simulink subsystem "Vehicle_Forces_Moments"  (R2025b)
settings: Solver=VariableStepAuto  StartTime=0.0  StopTime=10.0  RelTol=1e-3
undefined symbols (not defined in the file): ActTC
libraries: aerolibactuator x2
settings Model: Creator=cdriggs  LastModifiedBy=Ky Bui

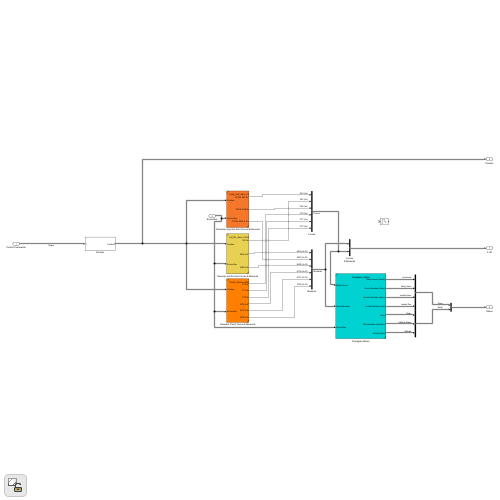
[thumbnail: Simulink's stored preview of the top-level diagram]
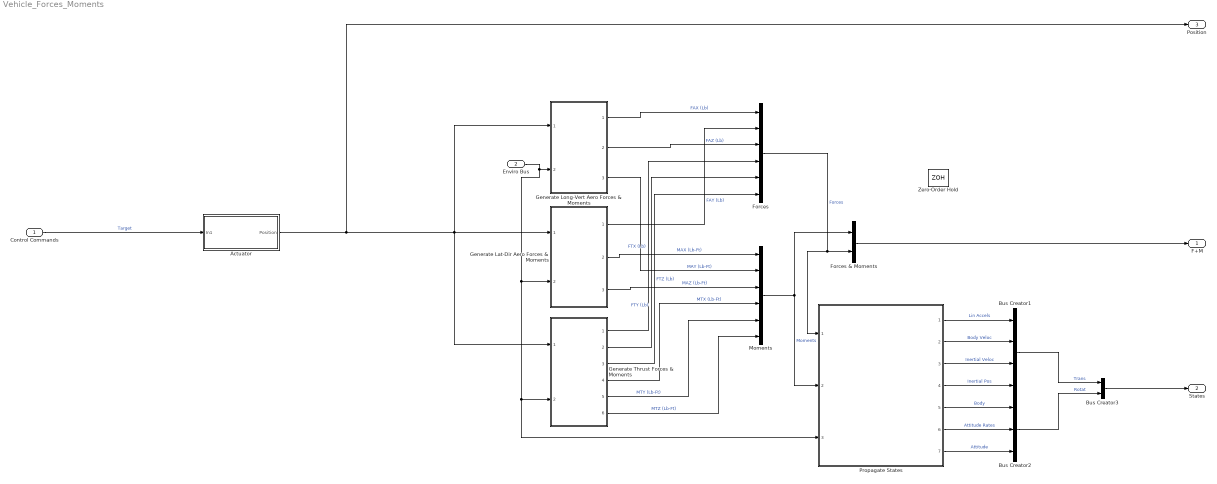
== system Vehicle_Forces_Moments ==
  Control Commands : Inport
  Enviro Bus : Inport  Port=2
  Actuator : Subsystem
  Bus Creator1 : BusCreator  Inputs=4
  Bus Creator2 : BusCreator  Inputs=3
  Bus Creator3 : BusCreator  Inputs=2
  Forces : BusCreator  Inputs=6
  Forces & Moments : BusCreator  Inputs=2
  Generate Lat-Dir Aero Forces & Moments : Subsystem  ReferencedSubsystem=Lat_Dir_Aero_Forces_Moments
  Generate Long-Vert Aero Forces & Moments : Subsystem  ReferencedSubsystem=Long_Vert_Aero_Forces_Moments
  Generate Thrust Forces & Moments : Subsystem  ReferencedSubsystem=Thrust_Forces_Moments
  Moments : BusCreator  Inputs=6
  Propagate States : Subsystem  ReferencedSubsystem=Propagate_States
  Zero-Order Hold : ZeroOrderHold  SampleTime=-1
  F+M : Outport
  States : Outport  Port=2
  Position : Outport  Port=3
  wires:
  Generate Lat-Dir Aero Forces & Moments/1 -> Forces/2  "FAY (Lb)"
  Generate Lat-Dir Aero Forces & Moments/2 -> Moments/1  "MAX (Lb-Ft)"
  Generate Lat-Dir Aero Forces & Moments/3 -> Moments/3  "MAZ (Lb-Ft)"
  Generate Thrust Forces & Moments/1 -> Forces/4  "FTX (Lb)"
  Generate Thrust Forces & Moments/2 -> Forces/5  "FTY (Lb)"
  Generate Thrust Forces & Moments/3 -> Forces/6  "FTZ (Lb)"
  Generate Thrust Forces & Moments/4 -> Moments/4  "MTX (Lb-Ft)"
  Generate Thrust Forces & Moments/5 -> Moments/5  "MTY (Lb-Ft)"
  Generate Thrust Forces & Moments/6 -> Moments/6  "MTZ (Lb-Ft)"
  Bus Creator2/1 -> Bus Creator3/2  "Rotat"
  Propagate States/4 -> Bus Creator1/4  "Inertial Pos"
  Bus Creator1/1 -> Bus Creator3/1  "Trans"
  Moments/1 -> Propagate States/2, Forces & Moments/1  "Moments"
  Propagate States/6 -> Bus Creator2/2  "Attitude Rates"
  Bus Creator3/1 -> States/1
  Propagate States/1 -> Bus Creator1/1  "Lin Accels"
  Forces & Moments/1 -> F+M/1
  Propagate States/3 -> Bus Creator1/3  "Inertial Veloc"
  Propagate States/5 -> Bus Creator2/1  "Body"
  Propagate States/7 -> Bus Creator2/3  "Attitude"
  Forces/1 -> Propagate States/1, Forces & Moments/2  "Forces"
  Generate Long-Vert Aero Forces & Moments/1 -> Forces/1  "FAX (Lb)"
  Generate Long-Vert Aero Forces & Moments/2 -> Forces/3  "FAZ (Lb)"
  Generate Long-Vert Aero Forces & Moments/3 -> Moments/2  "MAY (Lb-Ft)"
  Propagate States/2 -> Bus Creator1/2  "Body Veloc"
  Enviro Bus/1 -> Generate Long-Vert Aero Forces & Moments/2, Generate Lat-Dir Aero Forces & Moments/2, Generate Thrust Forces & Moments/2, Propagate States/3
  Actuator/1(Position) -> Generate Lat-Dir Aero Forces & Moments/1, Generate Thrust Forces & Moments/1, Generate Long-Vert Aero Forces & Moments/1, Position/1
  Control Commands/1 -> Actuator/1(In1)  "Target"

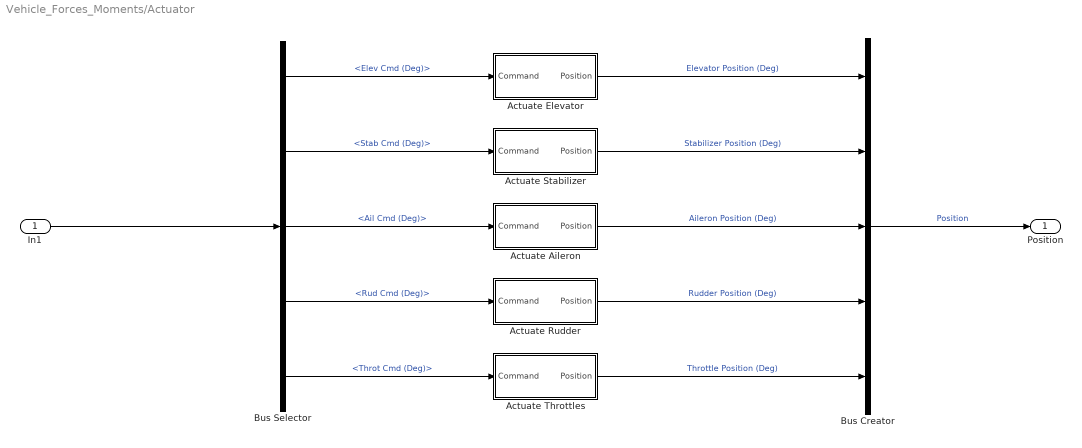
== system Vehicle_Forces_Moments/Actuator ==
  In1 : Inport
  Actuate Aileron : Subsystem
  Actuate Elevator : Subsystem
  Actuate Rudder : Subsystem
  Actuate Stabilizer : Subsystem
  Actuate Throttles : Subsystem
  Bus Creator : BusCreator  Inputs=5
  Bus Selector : BusSelector  OutputSignals=Elev Cmd (Deg),Stab Cmd (Deg),Ail Cmd (Deg),Rud Cmd (Deg),Throt Cmd (Deg)
  Position : Outport
  wires:
  Bus Creator/1 -> Position/1  "Position"
  In1/1 -> Bus Selector/1
  Bus Selector/2 -> Actuate Stabilizer/1(Command)  "<Stab Cmd (Deg)>"
  Actuate Stabilizer/1(Position) -> Bus Creator/2  "Stabilizer Position (Deg)"
  Actuate Throttles/1(Position) -> Bus Creator/5  "Throttle Position (Deg)"
  Actuate Rudder/1(Position) -> Bus Creator/4  "Rudder Position (Deg)"
  Bus Selector/5 -> Actuate Throttles/1(Command)  "<Throt Cmd (Deg)>"
  Bus Selector/3 -> Actuate Aileron/1(Command)  "<Ail Cmd (Deg)>"
  Actuate Aileron/1(Position) -> Bus Creator/3  "Aileron Position (Deg)"
  Bus Selector/4 -> Actuate Rudder/1(Command)  "<Rud Cmd (Deg)>"
  Bus Selector/1 -> Actuate Elevator/1(Command)  "<Elev Cmd (Deg)>"
  Actuate Elevator/1(Position) -> Bus Creator/1  "Elevator Position (Deg)"

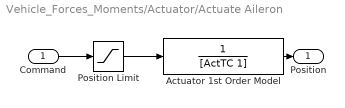
== system Vehicle_Forces_Moments/Actuator/Actuate Aileron ==
  Command : Inport
  Actuator 1st Order Model : TransferFcn  Denominator=[ActTC 1]
  Position Limit : Saturate  UpperLimit=30  LowerLimit=-30
  Position : Outport
  wires:
  Actuator 1st Order Model/1 -> Position/1
  Position Limit/1 -> Actuator 1st Order Model/1
  Command/1 -> Position Limit/1

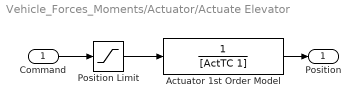
== system Vehicle_Forces_Moments/Actuator/Actuate Elevator ==
  Command : Inport
  Actuator 1st Order Model : TransferFcn  Denominator=[ActTC 1]
  Position Limit : Saturate  UpperLimit=30  LowerLimit=-30
  Position : Outport
  wires:
  Actuator 1st Order Model/1 -> Position/1
  Position Limit/1 -> Actuator 1st Order Model/1
  Command/1 -> Position Limit/1

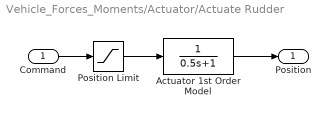
== system Vehicle_Forces_Moments/Actuator/Actuate Rudder ==
  Command : Inport
  Actuator 1st Order Model : TransferFcn  Denominator=[0.5 1]
  Position Limit : Saturate  UpperLimit=30  LowerLimit=-30
  Position : Outport
  wires:
  Actuator 1st Order Model/1 -> Position/1
  Position Limit/1 -> Actuator 1st Order Model/1
  Command/1 -> Position Limit/1

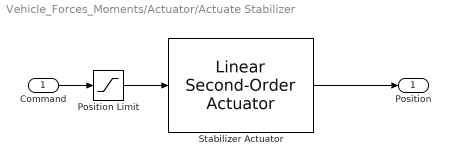
== system Vehicle_Forces_Moments/Actuator/Actuate Stabilizer ==
  Command : Inport
  Position Limit : Saturate  UpperLimit=15  LowerLimit=-5
  Stabilizer Actuator : aerolibactuator/Linear Second-Order Actuator  wn_fin=0.3  z_fin=1.0  fin_act_0=StabTrimPos  fin_act_vel=0
  Position : Outport
  wires:
  Command/1 -> Position Limit/1
  Position Limit/1 -> Stabilizer Actuator/1
  Stabilizer Actuator/1 -> Position/1

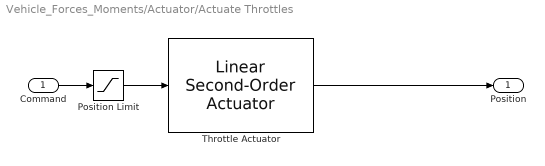
== system Vehicle_Forces_Moments/Actuator/Actuate Throttles ==
  Command : Inport
  Position Limit : Saturate  UpperLimit=1  LowerLimit=0
  Throttle Actuator : aerolibactuator/Linear Second-Order Actuator  wn_fin=1  z_fin=1.0  fin_act_0=EngineThrustCMD  fin_act_vel=0
  Position : Outport
  wires:
  Position Limit/1 -> Throttle Actuator/1
  Command/1 -> Position Limit/1
  Throttle Actuator/1 -> Position/1
